simulink model "linealidad"  (R2018a)
settings: Solver=VariableStepAuto  StartTime=0.0  StopTime=10.0  MaxStep=1e-2  RelTol=1e-3
settings Model: Creator=carma  LastModifiedBy=carma

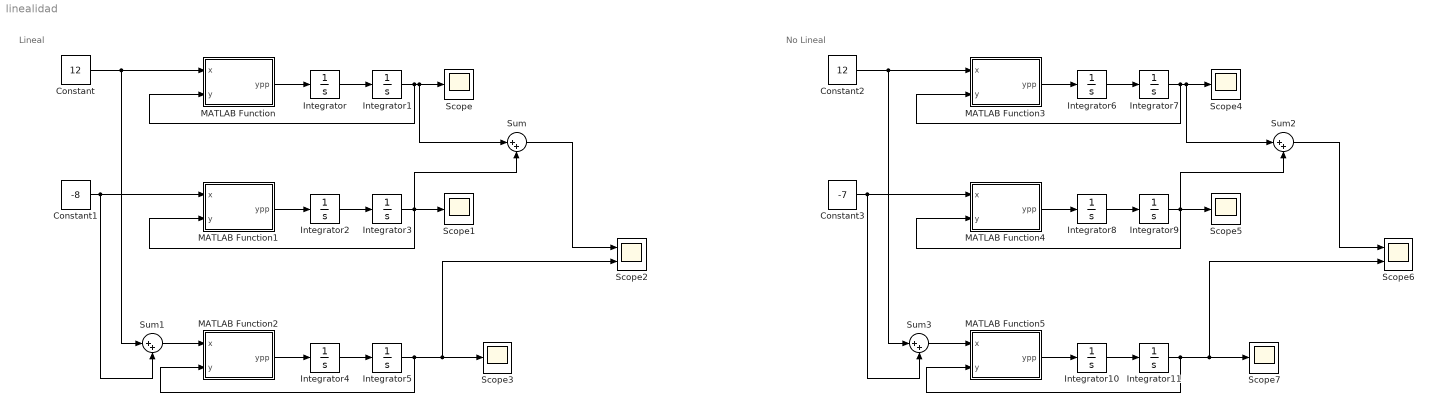
== system linealidad ==
  note: Lineal
  note: No Lineal
  Constant : Constant  Value=12
  Constant1 : Constant  Value=-8
  Constant2 : Constant  Value=12
  Constant3 : Constant  Value=-7
  Integrator{,1..11} (12 alike) : Integrator
  MATLAB Function : MATLAB Function  TreatAsAtomicUnit=on
  MATLAB Function1 : MATLAB Function  TreatAsAtomicUnit=on
  MATLAB Function2 : MATLAB Function  TreatAsAtomicUnit=on
  MATLAB Function3 : MATLAB Function  TreatAsAtomicUnit=on
  MATLAB Function4 : MATLAB Function  TreatAsAtomicUnit=on
  MATLAB Function5 : MATLAB Function  TreatAsAtomicUnit=on
  Scope{,1,3..5,7} (6 alike) : Scope
  Scope2 : Scope  NumInputPorts=2
  Scope6 : Scope  NumInputPorts=2
  Sum{,1..3} (4 alike) : Sum  Inputs=|++
  wires:
  MATLAB Function/1(ypp) -> Integrator/1
  Integrator/1 -> Integrator1/1
  Integrator1/1 -> MATLAB Function/2(y), Sum/1, Scope/1
  Constant/1 -> Sum1/1, MATLAB Function/1(x)
  Constant1/1 -> Sum1/2, MATLAB Function1/1(x)
  MATLAB Function1/1(ypp) -> Integrator2/1
  Integrator2/1 -> Integrator3/1
  Integrator3/1 -> Sum/2, MATLAB Function1/2(y), Scope1/1
  Sum/1 -> Scope2/1
  Sum1/1 -> MATLAB Function2/1(x)
  MATLAB Function2/1(ypp) -> Integrator4/1
  Integrator4/1 -> Integrator5/1
  Integrator5/1 -> MATLAB Function2/2(y), Scope3/1, Scope2/2
  Integrator10/1 -> Integrator11/1
  MATLAB Function5/1(ypp) -> Integrator10/1
  Sum2/1 -> Scope6/1
  Sum3/1 -> MATLAB Function5/1(x)
  Constant2/1 -> Sum3/1, MATLAB Function3/1(x)
  Integrator9/1 -> Sum2/2, MATLAB Function4/2(y), Scope5/1
  Integrator8/1 -> Integrator9/1
  Constant3/1 -> Sum3/2, MATLAB Function4/1(x)
  MATLAB Function4/1(ypp) -> Integrator8/1
  MATLAB Function3/1(ypp) -> Integrator6/1
  Integrator6/1 -> Integrator7/1
  Integrator7/1 -> MATLAB Function3/2(y), Sum2/1, Scope4/1
  Integrator11/1 -> MATLAB Function5/2(y), Scope7/1, Scope6/2

== matlab function linealidad/MATLAB Function1 ==
  data: x input; ypp output; y input
function ypp = fcn(x,y)
%#codegen

ypp = (5*x-5*y)/3;

== matlab function linealidad/MATLAB Function ==
  data: x input; ypp output; y input
function ypp = fcn(x,y)
%#codegen

ypp = (5*x-5*y)/3;

== matlab function linealidad/MATLAB Function2 ==
  data: x input; ypp output; y input
function ypp = fcn(x,y)
%#codegen

ypp = (5*x-5*y)/3;

== matlab function linealidad/MATLAB Function3 ==
  data: x input; ypp output; y input
function ypp = fcn(x,y)
%#codegen

ypp = (5*x-5*y+4)/3;

== matlab function linealidad/MATLAB Function4 ==
  data: x input; ypp output; y input
function ypp = fcn(x,y)
%#codegen

ypp = (5*x-5*y+4)/3;

== matlab function linealidad/MATLAB Function5 ==
  data: x input; ypp output; y input
function ypp = fcn(x,y)
%#codegen

ypp = (5*x-5*y+4)/3;
